simulink model "vga_controller"  (R2020a)
settings: Solver=VariableStepAuto  StartTime=0.0  StopTime=10.0  RelTol=1e-3
libraries: simulink_extras x26
settings Model: SnapshotBufferSize=100  EnablePacing=on  PacingRate=0.001000  Creator=kishan  LastModifiedBy=kishan

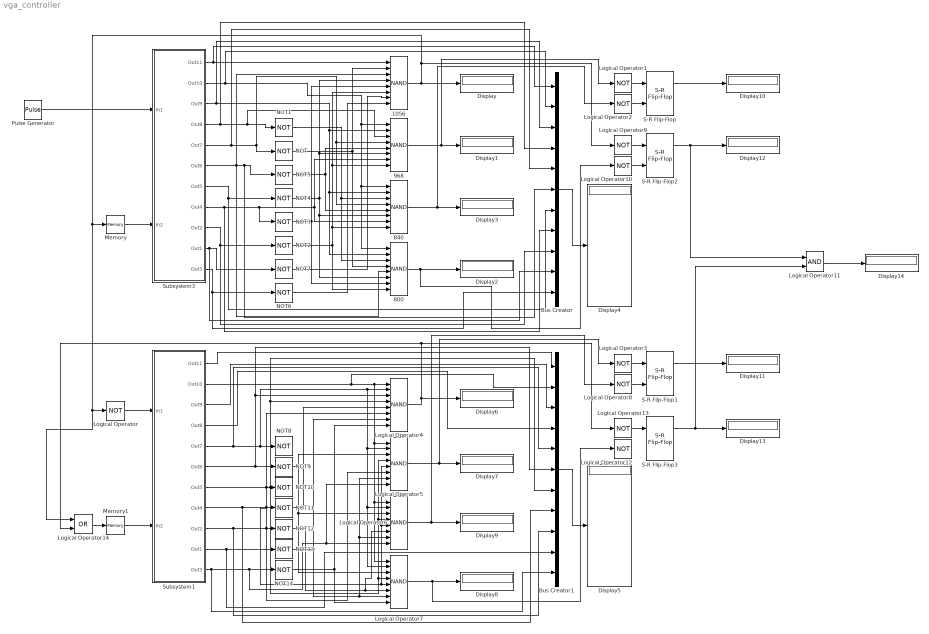
== system vga_controller ==
  {800,840,968,1056} (4 alike) : Logic  Operator=NAND  Inputs=8  AllPortsSameDT=off  OutDataTypeStr=boolean
  Bus Creator : BusCreator  Inputs=11
  Bus Creator1 : BusCreator  Inputs=11
  Display{,1..14} (15 alike) : Display
  Logical Operator : Logic  Operator=NOT  AllPortsSameDT=off  OutDataTypeStr=boolean
  Logical Operator{1..3,8..10,12..13} (8 alike) : Logic  Operator=NOT  IconShape=distinctive  AllPortsSameDT=off  OutDataTypeStr=boolean
  Logical Operator11 : Logic  AllPortsSameDT=off  OutDataTypeStr=boolean
  Logical Operator14 : Logic  Operator=OR  AllPortsSameDT=off  OutDataTypeStr=boolean
  Logical Operator{4..7} (4 alike) : Logic  Operator=NAND  Inputs=8  AllPortsSameDT=off  OutDataTypeStr=boolean
  Memory : Memory
  Memory1 : Memory
  NOT{,1..14} (15 alike) : Logic  Operator=NOT  IconShape=distinctive  AllPortsSameDT=off  OutDataTypeStr=boolean
  Pulse Generator : DiscretePulseGenerator  PulseType=Time based  Period=0.0000001  PulseWidth=5
  S-R Flip-Flop{,1..3} (4 alike) : simulink_extras/Flip Flops/S-R Flip-Flop  initial_condition=0
  Subsystem1 : Subsystem
  Subsystem3 : Subsystem
  wires:
  Subsystem3/2(Out10) -> Bus Creator/2, 968/1, 800/1, 840/1
  Subsystem3/3(Out9) -> Bus Creator/3, 968/2, 840/2, 800/2
  Subsystem3/9(Out2) -> Bus Creator/9, NOT2/1
  Subsystem3/8(Out4) -> Bus Creator/8, NOT3/1, 968/7, 840/7
  Subsystem3/7(Out5) -> Bus Creator/7, NOT4/1
  Subsystem3/4(Out8) -> Bus Creator/4, 968/3, NOT1/1
  Subsystem3/5(Out7) -> Bus Creator/5, NOT/1, 968/4, 840/4
  NOT1/1 -> 800/3, 840/3
  NOT/1 -> 1056/2, 800/4
  Subsystem3/6(Out6) -> Bus Creator/6, NOT5/1, 800/5, 1056/3
  NOT4/1 -> 968/6, 1056/4, 800/6, 840/6
  NOT3/1 -> 800/7, 1056/5
  NOT2/1 -> 968/8, 1056/6, 840/8, 800/8
  NOT5/1 -> 968/5, 840/5
  Subsystem3/1(Out11) -> Bus Creator/1, 1056/1
  Subsystem3/10(Out1) -> Bus Creator/10, NOT7/1
  Subsystem3/11(Out3) -> Bus Creator/11, NOT6/1
  NOT7/1 -> 1056/7
  NOT6/1 -> 1056/8
  1056/1 -> Logical Operator9/1, Logical Operator14/1, Logical Operator/1, Memory/1, Display/1
  Pulse Generator/1 -> Subsystem3/1(In1)
  968/1 -> Logical Operator1/1, Display1/1
  800/1 -> Logical Operator10/1, Display2/1
  840/1 -> Logical Operator2/1, Display3/1
  Bus Creator/1 -> Display4/1
  Memory/1 -> Subsystem3/2(In2)
  Logical Operator/1 -> Subsystem1/1(In1)
  Memory1/1 -> Subsystem1/2(In2)
  Subsystem1/2(Out10) -> Bus Creator1/2, Logical Operator7/1, Logical Operator6/1, Logical Operator5/1, Logical Operator4/1
  Subsystem1/5(Out7) -> Bus Creator1/5, NOT8/1, Logical Operator6/2, Logical Operator7/2, Logical Operator5/2, Logical Operator4/2
  Subsystem1/6(Out6) -> NOT9/1, Bus Creator1/6, Logical Operator4/3
  Subsystem1/7(Out5) -> Bus Creator1/7, Logical Operator4/4, Logical Operator5/4, Logical Operator6/4, Logical Operator7/4, NOT10/1
  Subsystem1/8(Out4) -> Bus Creator1/8, Logical Operator5/5, Logical Operator6/5, Logical Operator7/5, NOT11/1
  Subsystem1/9(Out2) -> Bus Creator1/9, Logical Operator4/6, NOT12/1, Logical Operator5/6
  Subsystem1/10(Out1) -> Bus Creator1/10, NOT13/1
  Subsystem1/11(Out3) -> Bus Creator1/11, Logical Operator6/8, Logical Operator5/8, NOT14/1
  NOT14/1 -> Logical Operator7/8, Logical Operator4/8
  NOT13/1 -> Logical Operator7/7, Logical Operator6/7, Logical Operator5/7, Logical Operator4/7
  NOT11/1 -> Logical Operator4/5
  NOT9/1 -> Logical Operator6/3, Logical Operator7/3, Logical Operator5/3
  NOT12/1 -> Logical Operator6/6, Logical Operator7/6
  Bus Creator1/1 -> Display5/1
  Subsystem1/1(Out11) -> Bus Creator1/1
  Subsystem1/3(Out9) -> Bus Creator1/3
  Subsystem1/4(Out8) -> Bus Creator1/4
  Logical Operator4/1 -> Logical Operator14/2, Logical Operator13/1, Display6/1
  Logical Operator7/1 -> Logical Operator12/1, Display8/1
  S-R Flip-Flop/1 -> Display10/1
  Logical Operator2/1 -> S-R Flip-Flop/2
  Logical Operator1/1 -> S-R Flip-Flop/1
  Logical Operator8/1 -> S-R Flip-Flop1/2
  Logical Operator5/1 -> Logical Operator3/1, Display7/1
  Logical Operator3/1 -> S-R Flip-Flop1/1
  Logical Operator6/1 -> Logical Operator8/1, Display9/1
  S-R Flip-Flop1/1 -> Display11/1
  Logical Operator9/1 -> S-R Flip-Flop2/1
  Logical Operator10/1 -> S-R Flip-Flop2/2
  S-R Flip-Flop2/1 -> Logical Operator11/1, Display12/1
  S-R Flip-Flop3/1 -> Logical Operator11/2, Display13/1
  Logical Operator13/1 -> S-R Flip-Flop3/1
  Logical Operator14/1 -> Memory1/1
  Logical Operator11/1 -> Display14/1

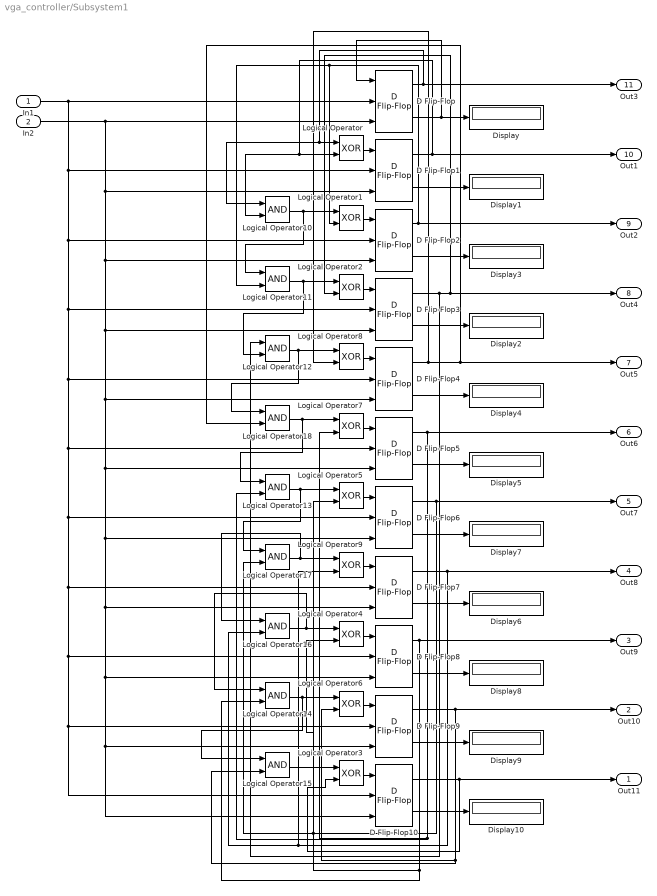
== system vga_controller/Subsystem1 ==
  In1 : Inport
  In2 : Inport  Port=2
  D Flip-Flop{,1..10} (11 alike) : simulink_extras/Flip Flops/D Flip-Flop
  Display{,1..10} (11 alike) : Display
  Logical Operator{,1..9} (10 alike) : Logic  Operator=XOR  AllPortsSameDT=off  OutDataTypeStr=boolean
  Logical Operator{10..18} (9 alike) : Logic  AllPortsSameDT=off  OutDataTypeStr=boolean
  Out11 : Outport
  Out10 : Outport  Port=2
  Out9 : Outport  Port=3
  Out8 : Outport  Port=4
  Out7 : Outport  Port=5
  Out6 : Outport  Port=6
  Out5 : Outport  Port=7
  Out4 : Outport  Port=8
  Out2 : Outport  Port=9
  Out1 : Outport  Port=10
  Out3 : Outport  Port=11
  wires:
  D Flip-Flop9/2 -> Display9/1
  D Flip-Flop4/2 -> Display4/1
  D Flip-Flop6/2 -> Display7/1
  D Flip-Flop5/2 -> Display5/1
  D Flip-Flop2/1 -> Logical Operator11/2, Logical Operator1/2, Out2/1
  D Flip-Flop3/1 -> Logical Operator12/1, Logical Operator2/2, Out4/1
  D Flip-Flop8/1 -> Logical Operator14/2, Logical Operator4/2, Out9/1
  D Flip-Flop3/2 -> Display2/1
  D Flip-Flop2/2 -> Display3/1
  D Flip-Flop5/1 -> Logical Operator13/2, Logical Operator7/2, Out6/1
  D Flip-Flop8/2 -> Display8/1
  D Flip-Flop1/2 -> Display1/1
  D Flip-Flop7/2 -> Display6/1
  D Flip-Flop4/1 -> Logical Operator8/2, Logical Operator18/2, Out5/1
  D Flip-Flop7/1 -> Logical Operator16/2, Logical Operator9/2, Out8/1
  D Flip-Flop9/1 -> Logical Operator15/2, Logical Operator6/2, Out10/1
  D Flip-Flop/1 -> Logical Operator10/1, Logical Operator/1, Out3/1
  D Flip-Flop6/1 -> Logical Operator17/2, Logical Operator5/2, Out7/1
  D Flip-Flop1/1 -> Logical Operator10/2, Logical Operator/2, Out1/1
  D Flip-Flop/2 -> D Flip-Flop/1, Display/1
  D Flip-Flop10/2 -> Display10/1
  D Flip-Flop10/1 -> Out11/1, Logical Operator3/2
  Logical Operator/1 -> D Flip-Flop1/1
  Logical Operator1/1 -> D Flip-Flop2/1
  Logical Operator2/1 -> D Flip-Flop3/1
  Logical Operator3/1 -> D Flip-Flop10/1
  Logical Operator4/1 -> D Flip-Flop8/1
  Logical Operator5/1 -> D Flip-Flop6/1
  Logical Operator6/1 -> D Flip-Flop9/1
  Logical Operator7/1 -> D Flip-Flop5/1
  Logical Operator8/1 -> D Flip-Flop4/1
  Logical Operator9/1 -> D Flip-Flop7/1
  Logical Operator10/1 -> Logical Operator11/1, Logical Operator1/1
  Logical Operator11/1 -> Logical Operator12/2, Logical Operator2/1
  Logical Operator12/1 -> Logical Operator18/1, Logical Operator8/1
  Logical Operator13/1 -> Logical Operator17/1, Logical Operator5/1
  Logical Operator14/1 -> Logical Operator15/1, Logical Operator6/1
  Logical Operator15/1 -> Logical Operator3/1
  Logical Operator16/1 -> Logical Operator14/1, Logical Operator4/1
  Logical Operator17/1 -> Logical Operator16/1, Logical Operator9/1
  Logical Operator18/1 -> Logical Operator13/1, Logical Operator7/1
  In1/1 -> D Flip-Flop10/2, D Flip-Flop9/2, D Flip-Flop8/2, D Flip-Flop7/2, D Flip-Flop6/2, D Flip-Flop5/2, D Flip-Flop4/2, D Flip-Flop3/2, D Flip-Flop2/2, D Flip-Flop1/2, D Flip-Flop/2
  In2/1 -> D Flip-Flop10/3, D Flip-Flop9/3, D Flip-Flop8/3, D Flip-Flop7/3, D Flip-Flop6/3, D Flip-Flop5/3, D Flip-Flop4/3, D Flip-Flop3/3, D Flip-Flop2/3, D Flip-Flop1/3, D Flip-Flop/3

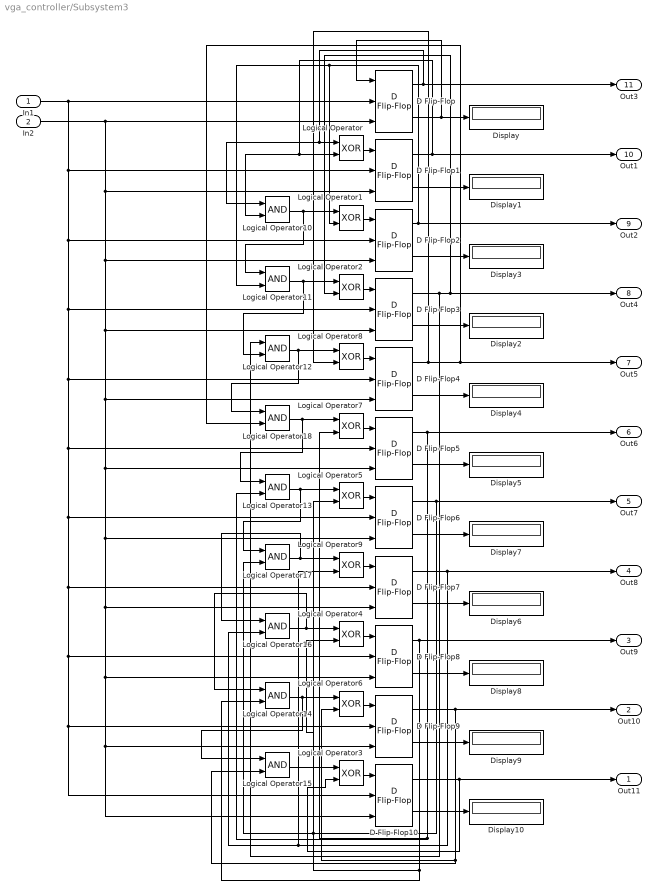
== system vga_controller/Subsystem3 ==
  In1 : Inport
  In2 : Inport  Port=2
  D Flip-Flop{,1..10} (11 alike) : simulink_extras/Flip Flops/D Flip-Flop
  Display{,1..10} (11 alike) : Display
  Logical Operator{,1..9} (10 alike) : Logic  Operator=XOR  AllPortsSameDT=off  OutDataTypeStr=boolean
  Logical Operator{10..18} (9 alike) : Logic  AllPortsSameDT=off  OutDataTypeStr=boolean
  Out11 : Outport
  Out10 : Outport  Port=2
  Out9 : Outport  Port=3
  Out8 : Outport  Port=4
  Out7 : Outport  Port=5
  Out6 : Outport  Port=6
  Out5 : Outport  Port=7
  Out4 : Outport  Port=8
  Out2 : Outport  Port=9
  Out1 : Outport  Port=10
  Out3 : Outport  Port=11
  wires:
  D Flip-Flop9/2 -> Display9/1
  D Flip-Flop4/2 -> Display4/1
  D Flip-Flop6/2 -> Display7/1
  D Flip-Flop5/2 -> Display5/1
  D Flip-Flop2/1 -> Logical Operator11/2, Logical Operator1/2, Out2/1
  D Flip-Flop3/1 -> Logical Operator12/1, Logical Operator2/2, Out4/1
  D Flip-Flop8/1 -> Logical Operator14/2, Logical Operator4/2, Out9/1
  D Flip-Flop3/2 -> Display2/1
  D Flip-Flop2/2 -> Display3/1
  D Flip-Flop5/1 -> Logical Operator13/2, Logical Operator7/2, Out6/1
  D Flip-Flop8/2 -> Display8/1
  D Flip-Flop1/2 -> Display1/1
  D Flip-Flop7/2 -> Display6/1
  D Flip-Flop4/1 -> Logical Operator8/2, Logical Operator18/2, Out5/1
  D Flip-Flop7/1 -> Logical Operator16/2, Logical Operator9/2, Out8/1
  D Flip-Flop9/1 -> Logical Operator15/2, Logical Operator6/2, Out10/1
  D Flip-Flop/1 -> Logical Operator10/1, Logical Operator/1, Out3/1
  D Flip-Flop6/1 -> Logical Operator17/2, Logical Operator5/2, Out7/1
  D Flip-Flop1/1 -> Logical Operator10/2, Logical Operator/2, Out1/1
  D Flip-Flop/2 -> D Flip-Flop/1, Display/1
  D Flip-Flop10/2 -> Display10/1
  D Flip-Flop10/1 -> Out11/1, Logical Operator3/2
  Logical Operator/1 -> D Flip-Flop1/1
  Logical Operator1/1 -> D Flip-Flop2/1
  Logical Operator2/1 -> D Flip-Flop3/1
  Logical Operator3/1 -> D Flip-Flop10/1
  Logical Operator4/1 -> D Flip-Flop8/1
  Logical Operator5/1 -> D Flip-Flop6/1
  Logical Operator6/1 -> D Flip-Flop9/1
  Logical Operator7/1 -> D Flip-Flop5/1
  Logical Operator8/1 -> D Flip-Flop4/1
  Logical Operator9/1 -> D Flip-Flop7/1
  Logical Operator10/1 -> Logical Operator11/1, Logical Operator1/1
  Logical Operator11/1 -> Logical Operator12/2, Logical Operator2/1
  Logical Operator12/1 -> Logical Operator18/1, Logical Operator8/1
  Logical Operator13/1 -> Logical Operator17/1, Logical Operator5/1
  Logical Operator14/1 -> Logical Operator15/1, Logical Operator6/1
  Logical Operator15/1 -> Logical Operator3/1
  Logical Operator16/1 -> Logical Operator14/1, Logical Operator4/1
  Logical Operator17/1 -> Logical Operator16/1, Logical Operator9/1
  Logical Operator18/1 -> Logical Operator13/1, Logical Operator7/1
  In1/1 -> D Flip-Flop10/2, D Flip-Flop9/2, D Flip-Flop8/2, D Flip-Flop7/2, D Flip-Flop6/2, D Flip-Flop5/2, D Flip-Flop4/2, D Flip-Flop3/2, D Flip-Flop2/2, D Flip-Flop1/2, D Flip-Flop/2
  In2/1 -> D Flip-Flop10/3, D Flip-Flop9/3, D Flip-Flop8/3, D Flip-Flop7/3, D Flip-Flop6/3, D Flip-Flop5/3, D Flip-Flop4/3, D Flip-Flop3/3, D Flip-Flop2/3, D Flip-Flop1/3, D Flip-Flop/3
